simulink model "torch_pos_with_sensors_tuning(1)"  (R2024a)
settings: Solver=FixedStepAuto  StartTime=0.0  StopTime=50  FixedStep=framePeriod_s  RelTol=1e-3
undefined symbols (not defined in the file): Aircraft, DiscIntNeverNeededParam, framePeriod_s, frameRate_hz, magnitude
libraries: simulink x37, slpidlib x10, simulink_extras x2, dspmathops x1
(part 4 of 4)

== matlab function torch_pos_with_sensors_tuning(1)/command selection/mode_norm/remap ==
  data: raw_in input; norm_out output; in_min input; in_max input; out_min input; out_max input
function norm_out = remap(raw_in,in_min,in_max,out_min,out_max)
norm_out = (raw_in - in_min) * (out_max - out_min)/(in_max-in_min) + out_min;
